simulink model "uz_codegen"  (R2021a)
settings: Solver=VariableStepAuto  StartTime=0.0  StopTime=0.1  RelTol=1e-3  EnableMultiTasking=on
PreLoadFcn:
  | uz_setCodegenPaths
model workspace (MATLAB code in the model file):
  | cmdLim = Simulink.Parameter;
  | cmdLim.Value = 15;
  | cmdLim.Description = 'Limit for controlling the maximum surface command angle.';
  | cmdLim.Min = 0;
  | cmdLim.Max = 90;
  | cmdLim.DocUnits = 'deg';
  | 
  | dispGain = Simulink.Parameter;
  | dispGain.Value = 0.75;
  | dispGain.Description = 'Gain applied to the displacement error.';
  | dispGain.Min = 0;
  | dispGain.Max = [];
  | dispGain.DocUnits = 'deg/sec/deg';
  | 
  | dispLim = Simulink.Parameter;
  | dispLim.Value = 30;
  | dispLim.Description = 'Limit for controlling the maximum commanded angle.';
  | dispLim.Min = 0;
  | dispLim.Max = 180;
  | dispLim.DocUnits = 'deg';
  | 
  | intGain = Simulink.Parameter;
  | intGain.Value = 0.5;
  | intGain.Description = 'Gain applied to the integral error.';
  | intGain.Min = 0;
  | intGain.Max = [];
  | intGain.DocUnits = 'deg/sec/deg/sec';
  | 
  | intLim = Simulink.Parameter;
  | intLim.Value = 5;
  | intLim.Description = 'Limit for controlling the maximum commanded angle.';
  | intLim.Min = 0;
  | intLim.Max = 90;
  | intLim.DocUnits = 'deg';
  | 
  | rateGain = Simulink.Parameter;
  | rateGain.Value = 2;
  | rateGain.Description = 'Gain applied to the rate error.';
  | rateGain.Min = 0;
  | rateGain.Max = [];
  | rateGain.DocUnits = 'deg/deg/sec';
  | 
  | rateLim = Simulink.Parameter;
  | rateLim.Value = 6;
  | rateLim.Description = 'Limit for controlling the maximum commanded angle.';
  | rateLim.Min = 0;
  | rateLim.Max = 180;
  | rateLim.DocUnits = 'deg/sec';
  | 
  | hdgGain = Simulink.Parameter;
  | hdgGain.Value = 0.015;
values from neighbouring files (symbols this model uses):
  f_switchingInverter = 20000    [PMSM_01_Parameter.m]
  Ki_IdController = Kp_IdController * Ki_IdController    (= 100.530964915)    [PMSM_01_Parameter.m]
  Ki_IqController = Kp_IqController * Ki_IqController    (= 100.530964915)    [PMSM_01_Parameter.m]
  Kp_IdController = Kp_IdController    (= 0.0402123859659)    [PMSM_01_Parameter.m]
  Kp_IqController = Kp_IqController    (= 0.0402123859659)    [PMSM_01_Parameter.m]
  Ld = Lq    (= 1.6e-05)    [PMSM_01_Parameter.m]
  Lq = 16e-6    (= 1.6e-05)    [PMSM_01_Parameter.m]
  psi_pm = 0.0048    [PMSM_01_Parameter.m]
  T_controller = 1/f_CurrentController    (= 5e-05)    [PMSM_01_Parameter.m]
  T_dead = 0.2e-10    (= 2e-11)    [PMSM_01_Parameter.m]
  U_DC = 46    [PMSM_01_Parameter.m]
  zp = 21    [PMSM_01_Parameter.m]
undefined symbols (not defined in the file or in its folder): DiscIntNeverNeededParam, U_maxDQ
libraries: nesl_utility x17, ee_lib x15, fl_lib x13, simulink x7, dspsrcs4 x3, pid_lib x2, spsTriangleGeneratorLib x1, spsabctodq0Lib x1, spsdq0toabcLib x1, spsdq0toAlphaBetaZeroLib x1, embmathops x1
(part 2 of 2)

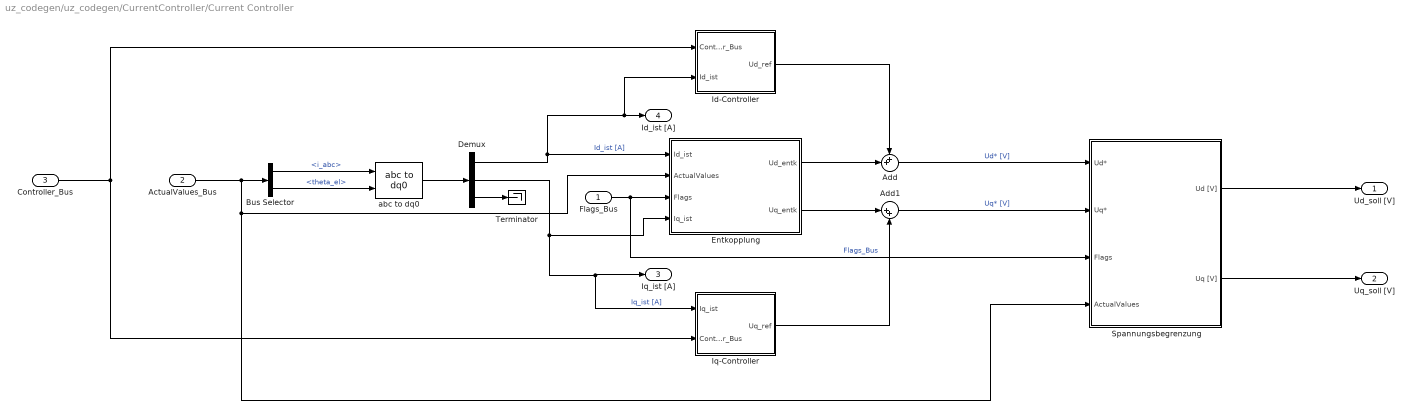
== system uz_codegen/uz_codegen/CurrentController/Current Controller ==
  Flags_Bus : Inport
  ActualValues_Bus : Inport  Port=2
  Controller_Bus : Inport  Port=3
  Add : Sum  Inputs=++|
  Add1 : Sum  Inputs=|++
  Bus Selector : BusSelector  OutputSignals=i_abc,theta_el
  Demux : Demux  Outputs=3
  Entkopplung : Subsystem
  Id-Controller : Subsystem
  Iq-Controller : Subsystem
  Spannungsbegrenzung : Subsystem
  Terminator : Terminator
  abc to dq0 : spsabctodq0Lib/abc to dq0  Alignment=Aligned with phase A axis
  Ud_soll [V] : Outport
  Uq_soll [V] : Outport  Port=2
  Iq_ist [A] : Outport  Port=3
  Id_ist [A] : Outport  Port=4
  wires:
  Add1/1 -> Spannungsbegrenzung/2(Uq*)  "Uq* [V]"
  Add/1 -> Spannungsbegrenzung/1(Ud*)  "Ud* [V]"
  abc to dq0/1 -> Demux/1
  Demux/1 -> Entkopplung/1(Id_ist), Id-Controller/2(Id_ist), Id_ist [A]/1  "Id_ist [A]"
  Demux/2 -> Entkopplung/4(Iq_ist), Iq_ist [A]/1, Iq-Controller/1(Iq_ist)  "Iq_ist [A]"
  Demux/3 -> Terminator/1
  Iq-Controller/1(Uq_ref) -> Add1/2
  Entkopplung/1(Ud_entk) -> Add/2
  Entkopplung/2(Uq_entk) -> Add1/1
  Id-Controller/1(Ud_ref) -> Add/1
  Spannungsbegrenzung/1(Ud [V]) -> Ud_soll [V]/1
  Spannungsbegrenzung/2(Uq [V]) -> Uq_soll [V]/1
  Controller_Bus/1 -> Id-Controller/1(Controller_Bus), Iq-Controller/2(Controller_Bus)
  Bus Selector/1 -> abc to dq0/1  "<i_abc>"
  Bus Selector/2 -> abc to dq0/2  "<theta_el>"
  ActualValues_Bus/1 -> Spannungsbegrenzung/4(ActualValues), Entkopplung/2(ActualValues), Bus Selector/1
  Flags_Bus/1 -> Spannungsbegrenzung/3(Flags), Entkopplung/3(Flags)  "Flags_Bus"

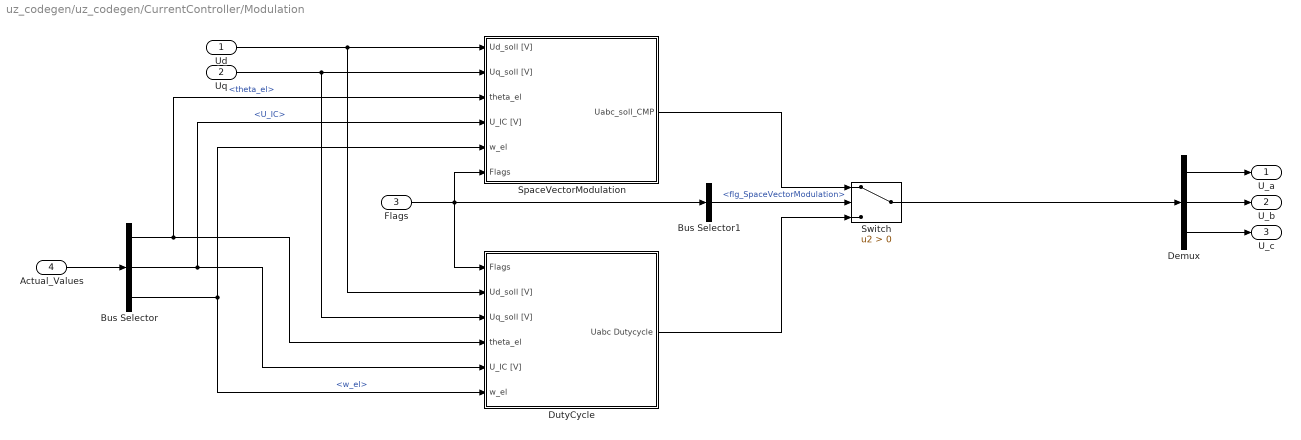
== system uz_codegen/uz_codegen/CurrentController/Modulation ==
  Ud : Inport
  Uq : Inport  Port=2
  Flags : Inport  Port=3
  Actual_Values : Inport  Port=4
  Bus Selector : BusSelector  OutputSignals=theta_el,U_IC,w_el
  Bus Selector1 : BusSelector  OutputSignals=flg_SpaceVectorModulation
  Demux : Demux  Outputs=3
  DutyCycle : Subsystem
  SpaceVectorModulation : Subsystem
  Switch : Switch  Criteria=u2 > Threshold
  U_a : Outport
  U_b : Outport  Port=2
  U_c : Outport  Port=3
  wires:
  Demux/2 -> U_b/1
  Bus Selector1/1 -> Switch/2  "<flg_SpaceVectorModulation>"
  Demux/3 -> U_c/1
  Demux/1 -> U_a/1
  Switch/1 -> Demux/1
  Ud/1 -> DutyCycle/2(Ud_soll [V]), SpaceVectorModulation/1(Ud_soll [V])
  Uq/1 -> DutyCycle/3(Uq_soll [V]), SpaceVectorModulation/2(Uq_soll [V])
  Actual_Values/1 -> Bus Selector/1
  Bus Selector/1 -> DutyCycle/4(theta_el), SpaceVectorModulation/3(theta_el)  "<theta_el>"
  Bus Selector/2 -> DutyCycle/5(U_IC [V]), SpaceVectorModulation/4(U_IC [V])  "<U_IC>"
  Bus Selector/3 -> DutyCycle/6(w_el), SpaceVectorModulation/5(w_el)  "<w_el>"
  DutyCycle/1(Uabc Dutycycle) -> Switch/3
  SpaceVectorModulation/1(Uabc_soll_CMP) -> Switch/1
  Flags/1 -> SpaceVectorModulation/6(Flags), DutyCycle/1(Flags), Bus Selector1/1

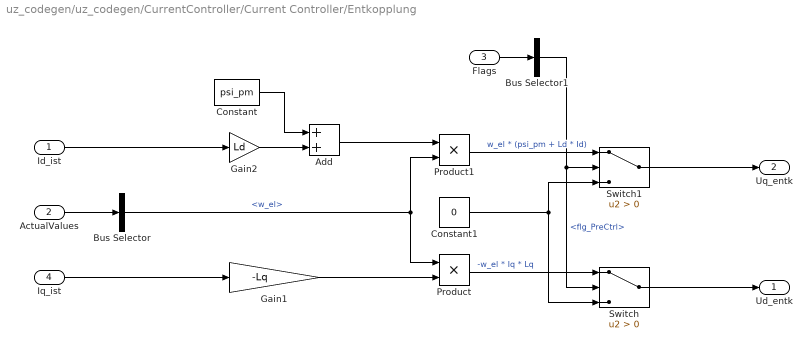
== system uz_codegen/uz_codegen/CurrentController/Current Controller/Entkopplung ==
  Id_ist : Inport
  ActualValues : Inport  Port=2
  Flags : Inport  Port=3
  Iq_ist : Inport  Port=4
  Add : Sum
  Bus Selector : BusSelector  OutputSignals=w_el
  Bus Selector1 : BusSelector  OutputSignals=flg_PreCtrl
  Constant : Constant  Value=psi_pm
  Constant1 : Constant  Value=0
  Gain1 : Gain  Gain=-Lq
  Gain2 : Gain  Gain=Ld
  Product : Product
  Product1 : Product
  Switch : Switch  Criteria=u2 > Threshold
  Switch1 : Switch  Criteria=u2 > Threshold
  Ud_entk : Outport
  Uq_entk : Outport  Port=2
  wires:
  Bus Selector/1 -> Product1/2, Product/1  "<w_el>"
  Iq_ist/1 -> Gain1/1
  Gain1/1 -> Product/2
  Product/1 -> Switch/1  "-w_el * Iq * Lq"
  Id_ist/1 -> Gain2/1
  Gain2/1 -> Add/2
  Constant/1 -> Add/1
  Add/1 -> Product1/1
  Product1/1 -> Switch1/1  "w_el * (psi_pm + Ld * Id)"
  Switch/1 -> Ud_entk/1
  Switch1/1 -> Uq_entk/1
  Constant1/1 -> Switch1/3, Switch/3
  Flags/1 -> Bus Selector1/1
  Bus Selector1/1 -> Switch1/2, Switch/2  "<flg_PreCtrl>"
  ActualValues/1 -> Bus Selector/1

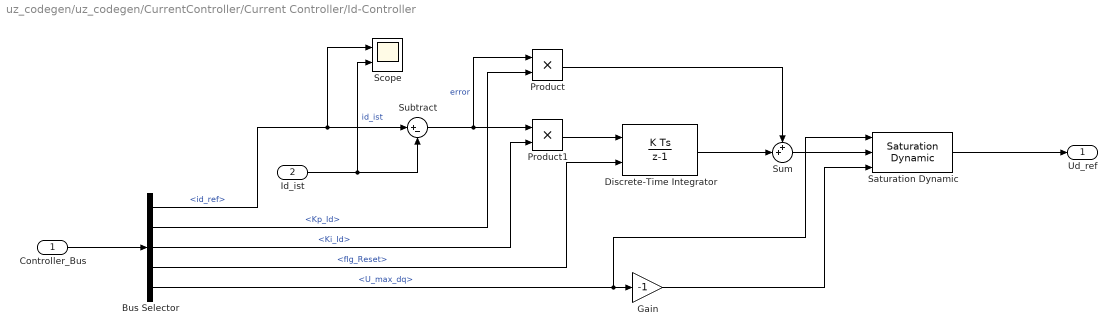
== system uz_codegen/uz_codegen/CurrentController/Current Controller/Id-Controller ==
  Controller_Bus : Inport
  Id_ist : Inport  Port=2
  Bus Selector : BusSelector  OutputSignals=id_ref,Kp_Id,Ki_Id,flg_Reset,U_max_dq
  Discrete-Time Integrator : DiscreteIntegrator  ExternalReset=level  SampleTime=-1  ICPrevOutput=DiscIntNeverNeededParam  ICPrevScaledInput=DiscIntNeverNeededParam
  Gain : Gain  Gain=-1
  Product : Product
  Product1 : Product
  Saturation Dynamic : simulink/Discontinuities/Saturation Dynamic  OutMin=[]  OutMax=[]  OutDataTypeStr=Inherit: Same as second input  OutDataType=fixdt(1, 16)  OutScaling=2^-10  DoSatur=off
  Scope : Scope  NumInputPorts=2
  Subtract : Sum  Inputs=|+-
  Sum : Sum  Inputs=++|
  Ud_ref : Outport
  wires:
  Bus Selector/1 -> Scope/1, Subtract/1  "<id_ref>"
  Gain/1 -> Saturation Dynamic/3
  Bus Selector/2 -> Product/2  "<Kp_Id>"
  Bus Selector/4 -> Discrete-Time Integrator/2  "<flg_Reset>"
  Id_ist/1 -> Subtract/2, Scope/2  "id_ist"
  Bus Selector/3 -> Product1/2  "<Ki_Id>"
  Controller_Bus/1 -> Bus Selector/1
  Bus Selector/5 -> Saturation Dynamic/1, Gain/1  "<U_max_dq>"
  Sum/1 -> Saturation Dynamic/2
  Saturation Dynamic/1 -> Ud_ref/1
  Product/1 -> Sum/1
  Subtract/1 -> Product/1, Product1/1  "error"
  Discrete-Time Integrator/1 -> Sum/2
  Product1/1 -> Discrete-Time Integrator/1

== system uz_codegen/uz_codegen/CurrentController/Current Controller/Iq-Controller ==
  Iq_ist : Inport
  Controller_Bus : Inport  Port=2
  Bus Selector : BusSelector  OutputSignals=iq_ref,Kp_Iq,Ki_Iq,flg_Reset,U_max_dq
  Discrete-Time Integrator : DiscreteIntegrator  ExternalReset=level  SampleTime=-1  ICPrevOutput=DiscIntNeverNeededParam  ICPrevScaledInput=DiscIntNeverNeededParam
  Gain : Gain  Gain=-1
  Product : Product
  Product1 : Product
  Saturation Dynamic : simulink/Discontinuities/Saturation Dynamic  OutMin=[]  OutMax=[]  OutDataTypeStr=Inherit: Same as second input  OutDataType=fixdt(1, 16)  OutScaling=2^-10  DoSatur=off
  Scope : Scope  NumInputPorts=2
  Subtract : Sum  Inputs=|+-
  Sum : Sum  Inputs=++|
  Uq_ref : Outport
  wires:
  Iq_ist/1 -> Subtract/2, Scope/2  "iq_ist"
  Controller_Bus/1 -> Bus Selector/1
  Bus Selector/2 -> Product/2  "<Kp_Iq>"
  Bus Selector/3 -> Product1/2  "<Ki_Iq>"
  Bus Selector/4 -> Discrete-Time Integrator/2  "<flg_Reset>"
  Bus Selector/5 -> Saturation Dynamic/1, Gain/1  "<U_max_dq>"
  Gain/1 -> Saturation Dynamic/3
  Bus Selector/1 -> Scope/1, Subtract/1  "<iq_ref>"
  Subtract/1 -> Product/1, Product1/1  "error"
  Product1/1 -> Discrete-Time Integrator/1
  Discrete-Time Integrator/1 -> Sum/2
  Product/1 -> Sum/1
  Sum/1 -> Saturation Dynamic/2
  Saturation Dynamic/1 -> Uq_ref/1

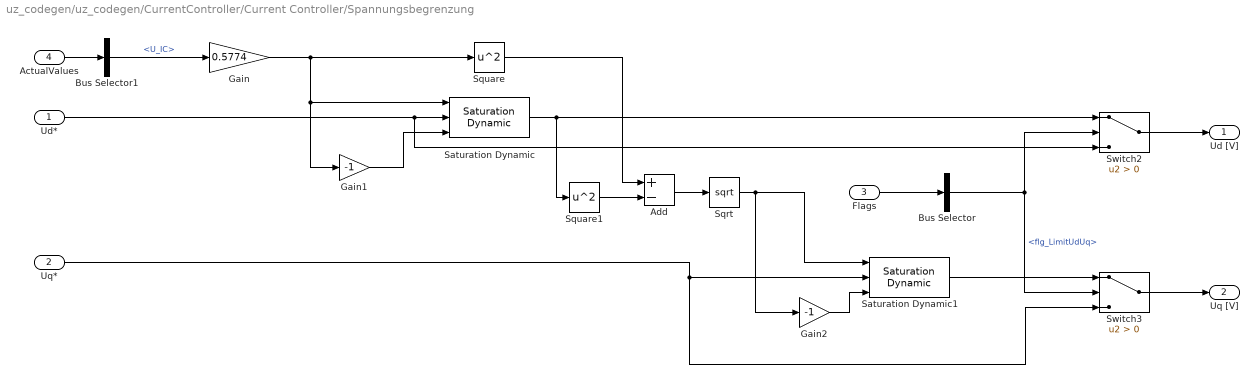
== system uz_codegen/uz_codegen/CurrentController/Current Controller/Spannungsbegrenzung ==
  Ud* : Inport
  Uq* : Inport  Port=2
  Flags : Inport  Port=3
  ActualValues : Inport  Port=4
  Add : Sum  Inputs=+-
  Bus Selector : BusSelector  OutputSignals=flg_LimitUdUq
  Bus Selector1 : BusSelector  OutputSignals=U_IC
  Gain : Gain  Gain=0.5774
  Gain1 : Gain  Gain=-1
  Gain2 : Gain  Gain=-1
  Saturation Dynamic : simulink/Discontinuities/Saturation Dynamic  OutMin=[]  OutMax=[]  OutDataTypeStr=Inherit: Same as second input  OutDataType=fixdt(1, 16)  OutScaling=2^-10  DoSatur=off
  Saturation Dynamic1 : simulink/Discontinuities/Saturation Dynamic  OutMin=[]  OutMax=[]  OutDataTypeStr=Inherit: Same as second input  OutDataType=fixdt(1, 16)  OutScaling=2^-10  DoSatur=off
  Sqrt : Sqrt  SaturateOnIntegerOverflow=on
  Square : Math  Operator=square  SaturateOnIntegerOverflow=on
  Square1 : Math  Operator=square  SaturateOnIntegerOverflow=on
  Switch2 : Switch  Criteria=u2 > Threshold
  Switch3 : Switch  Criteria=u2 > Threshold
  Ud [V] : Outport
  Uq [V] : Outport  Port=2
  wires:
  Gain2/1 -> Saturation Dynamic1/3
  Add/1 -> Sqrt/1
  Square/1 -> Add/1
  Sqrt/1 -> Gain2/1, Saturation Dynamic1/1
  Saturation Dynamic/1 -> Switch2/1, Square1/1
  Gain1/1 -> Saturation Dynamic/3
  Uq*/1 -> Saturation Dynamic1/2, Switch3/3
  Bus Selector1/1 -> Gain/1  "<U_IC>"
  Gain/1 -> Square/1, Saturation Dynamic/1, Gain1/1
  Square1/1 -> Add/2
  Ud*/1 -> Saturation Dynamic/2, Switch2/3
  Switch3/1 -> Uq [V]/1
  Switch2/1 -> Ud [V]/1
  Saturation Dynamic1/1 -> Switch3/1
  Flags/1 -> Bus Selector/1
  Bus Selector/1 -> Switch3/2, Switch2/2  "<flg_LimitUdUq>"
  ActualValues/1 -> Bus Selector1/1

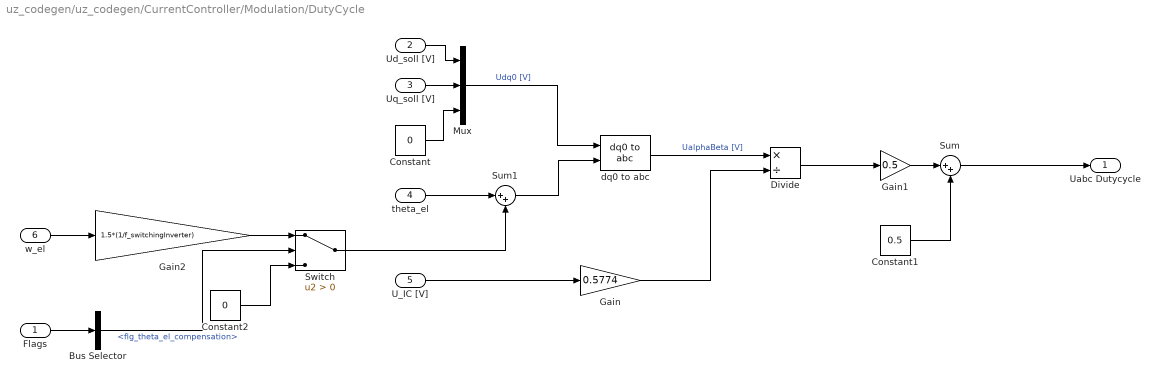
== system uz_codegen/uz_codegen/CurrentController/Modulation/DutyCycle ==
  Flags : Inport
  Ud_soll [V] : Inport  Port=2
  Uq_soll [V] : Inport  Port=3
  theta_el : Inport  Port=4
  U_IC [V] : Inport  Port=5
  w_el : Inport  Port=6
  Bus Selector : BusSelector  OutputSignals=flg_theta_el_compensation
  Constant : Constant  Value=0
  Constant1 : Constant  Value=0.5
  Constant2 : Constant  Value=0
  Divide : Product  Inputs=*/
  Gain : Gain  Gain=0.5774
  Gain1 : Gain  Gain=0.5
  Gain2 : Gain  Gain=1.5*(1/f_switchingInverter)
  Mux : Mux  Inputs=3
  Sum : Sum  Inputs=|++
  Sum1 : Sum  Inputs=|++
  Switch : Switch  Criteria=u2 > Threshold
  dq0 to abc : spsdq0toabcLib/dq0 to abc  Alignment=Aligned with phase A axis
  Uabc Dutycycle : Outport
  wires:
  Constant/1 -> Mux/3
  U_IC [V]/1 -> Gain/1
  dq0 to abc/1 -> Divide/1  "UalphaBeta [V]"
  Mux/1 -> dq0 to abc/1  "Udq0 [V]"
  Uq_soll [V]/1 -> Mux/2
  Ud_soll [V]/1 -> Mux/1
  theta_el/1 -> Sum1/1
  Gain/1 -> Divide/2
  Divide/1 -> Gain1/1
  Gain1/1 -> Sum/1
  Constant1/1 -> Sum/2
  Sum/1 -> Uabc Dutycycle/1
  Sum1/1 -> dq0 to abc/2
  w_el/1 -> Gain2/1
  Gain2/1 -> Switch/1
  Switch/1 -> Sum1/2
  Constant2/1 -> Switch/3
  Flags/1 -> Bus Selector/1
  Bus Selector/1 -> Switch/2  "<flg_theta_el_compensation>"

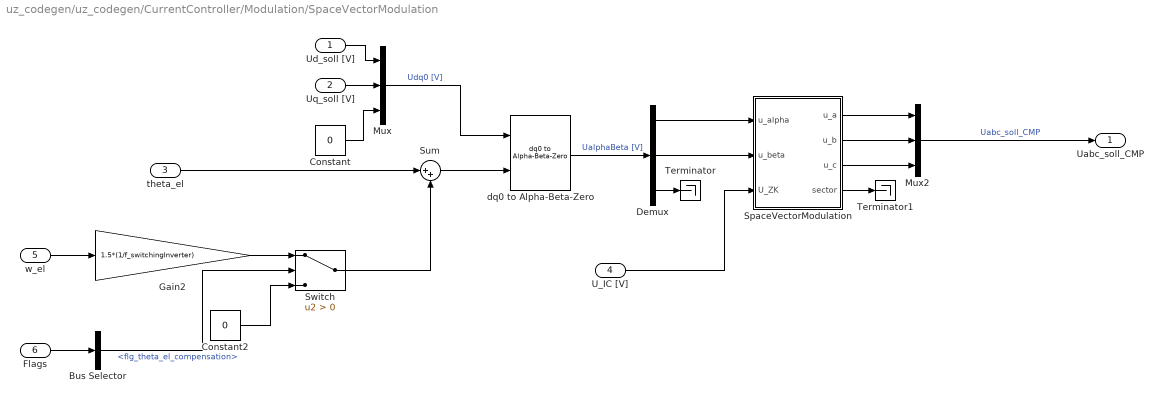
== system uz_codegen/uz_codegen/CurrentController/Modulation/SpaceVectorModulation ==
  Ud_soll [V] : Inport
  Uq_soll [V] : Inport  Port=2
  theta_el : Inport  Port=3
  U_IC [V] : Inport  Port=4
  w_el : Inport  Port=5
  Flags : Inport  Port=6
  Bus Selector : BusSelector  OutputSignals=flg_theta_el_compensation
  Constant : Constant  Value=0
  Constant2 : Constant  Value=0
  Demux : Demux  Outputs=3
  Gain2 : Gain  Gain=1.5*(1/f_switchingInverter)
  Mux : Mux  Inputs=3
  Mux2 : Mux  Inputs=3
  SpaceVectorModulation : MATLAB Function  TreatAsAtomicUnit=on
  Sum : Sum  Inputs=|++
  Switch : Switch  Criteria=u2 > Threshold
  Terminator : Terminator
  Terminator1 : Terminator
  dq0 to Alpha-Beta-Zero : spsdq0toAlphaBetaZeroLib/dq0 to Alpha-Beta-Zero  Alignment=Aligned with phase A axis
      settings: SourceProductBaseCode=PS
  Uabc_soll_CMP : Outport
  wires:
  Ud_soll [V]/1 -> Mux/1
  Uq_soll [V]/1 -> Mux/2
  Constant/1 -> Mux/3
  Mux/1 -> dq0 to Alpha-Beta-Zero/1  "Udq0 [V]"
  theta_el/1 -> Sum/1
  Demux/1 -> SpaceVectorModulation/1(u_alpha)
  Demux/2 -> SpaceVectorModulation/2(u_beta)
  Demux/3 -> Terminator/1
  SpaceVectorModulation/1(u_a) -> Mux2/1
  SpaceVectorModulation/2(u_b) -> Mux2/2
  SpaceVectorModulation/3(u_c) -> Mux2/3
  dq0 to Alpha-Beta-Zero/1 -> Demux/1  "UalphaBeta [V]"
  Mux2/1 -> Uabc_soll_CMP/1  "Uabc_soll_CMP"
  U_IC [V]/1 -> SpaceVectorModulation/3(U_ZK)
  SpaceVectorModulation/4(sector) -> Terminator1/1
  w_el/1 -> Gain2/1
  Constant2/1 -> Switch/3
  Flags/1 -> Bus Selector/1
  Gain2/1 -> Switch/1
  Bus Selector/1 -> Switch/2  "<flg_theta_el_compensation>"
  Sum/1 -> dq0 to Alpha-Beta-Zero/2
  Switch/1 -> Sum/2

== stateflow chart uz_codegen/uz_codegen ==
  settings: updateMethod=DISCRETE  sampleTime=T_controller
  state Start
    entry:
    activeState = 1;
    Ua_DutyCycle = 0;
    Ub_DutyCycle = 0;
    Uc_DutyCycle = 0;
  state Reset
    during:
    activeState = 3;
    [Ua_DutyCycle, Ub_DutyCycle, Uc_DutyCycle, iq_ist, id_ist, ud, uq] = CurrentController(ia, ib, ic, w_el, flg_PreCntr, theta_el, U_IC,id_ref,iq_ref,flgLimitUdUq, Kp_Iq, Ki_Iq, Kp_Id, Ki_Id, flg_SpaceVectorModulation, RESET, flg_deadTimeCompensation, flg_theta_el_compensation)
    Ua_DutyCycle = 0;
    Ub_DutyCycle = 0;
    Uc_DutyCycle = 0;
  state InProcess
    entry:
    activeState = 2;
    during:
    [Ua_DutyCycle, Ub_DutyCycle, Uc_DutyCycle, iq_ist, id_ist, ud, uq] = CurrentController(ia, ib, ic, w_el, flg_PreCntr, theta_el, U_IC,id_ref,iq_ref,flgLimitUdUq, Kp_Iq, Ki_Iq, Kp_Id, Ki_Id, flg_SpaceVectorModulation, RESET, flg_deadTimeCompensation, flg_theta_el_compensation)
  state [ua,ub,uc,Iq_ist,Id_ist,ud_soll,uq_soll] = CurrentController(ia,ib,ic,w_el,flg_PreCtrl,theta_el,U_IC,id_ref,iq_ref,flg_LimitUdUq,Kp_Iq,Ki_Iq,Kp_Id,Ki_Id,flg_SpaceVectorModulation,flg_Reset,flg_deadTimeCompensation, flg_theta_el_compensation) [function]
  (default) -> Start
  Reset -> Start : [RESET == 0]
  InProcess -> Reset : [RESET==1]
  Start -> InProcess : [START==1 & RESET==0]
  data: ia function_input double size=1; ib function_input double size=1; ic function_input double size=1; w_el function_input double size=1; flg_PreCtrl function_input double size=1; theta_el function_input double size=1; ua function_output; ub function_output; uc function_output; Iq_ist function_output; Id_ist function_output; ud_soll function_output; uq_soll function_output; U_IC function_input double size=1; id_ref function_input double size=1; iq_ref function_input double size=1; flg_LimitUdUq function_input double size=1; Kp_Iq function_input double size=1; Ki_Iq function_input double size=1; Kp_Id function_input double size=1; Ki_Id function_input double size=1; flg_SpaceVectorModulation function_input double size=1; flg_Reset function_input double size=1; flg_deadTimeCompensation function_input double size=1; flg_theta_el_compensation function_input double size=1; flg_PreCntr input; ic input; ib input; w_el input; ia input; theta_el input; iq_ref input; id_ref input; Ua_DutyCycle output; activeState output; Uc_DutyCycle output; Ub_DutyCycle output; iq_ist output; id_ist output; U_IC input; RESET input; START input; uq output; ud output; flgLimitUdUq input; flg_SpaceVectorModulation input; Kp_Iq input; Kp_Id input; Ki_Iq input; Ki_Id input; flg_deadTimeCompensation input; flg_theta_el_compensation input

== matlab function uz_codegen/CurrentController/Modulation/SpaceVectorModulation/SpaceVectorModulation ==
  data: u_alpha input; u_a output; u_beta input; U_ZK input; u_b output; u_c output; sector output
function [u_a, u_b, u_c, sector] = fcn(u_alpha, u_beta, U_ZK)

a_U_on=0;
a_V_on=0;
a_W_on=0;

 %%__%%__%%__%%__%%__%%__%%__%%__%%__%%__%%__%%__%%__%%__%%__%%__%%__%%__%%_
    %%Trägerbasierte Raumzeigermodulation%%
    %%Eingänge:
    %U_ZK       -- Zwischenkreisspannung
    %u_alpha    -- alphakomponente des Sollspannungsraumzeigers
    %u_beta     -- betakomponente des Sollspannungsraumzeigers
    %CMP_Period_max_val  -- maximalwert des Dreiecks/Sägezahnzählers zum Gewichten der Aussteuergrade
    %%Ausgänge:
    %CMP_U        -- Vergleichswert U
    %CMP_V        -- Vergleichswert V
    %CMP_W        -- Vergleichswert W
    %sector       -- Ausgabe des Sektors des Spannungszeigers
    
    
    %Berechnung von a, b, c nach Quang Dittrich S24
    
    a = abs(u_alpha) + 0.5774*abs(u_beta);
    b = abs(u_alpha) - 0.5774*abs(u_beta);
    c = 1.1547*abs(u_beta);
    
    U_max = 0.6667 * U_ZK; %Maximum Voltage U_ZL/sqrt(3)
    
    
    %Sektor und Quadranten nach Quang Dittrich S32
    if(u_beta < 0)
        if (u_alpha <0)
            quadrant=3;
            if(b < 0)
                sector = 5;
            else
                sector = 4;
            end
        else
            quadrant=4;
            if(b < 0)
                sector = 5;
            else
                sector = 6;
            end
        end
        
    else
        if (u_alpha <0)
            quadrant=2;
            if(b < 0)
                sector = 2;
            else
                sector = 3;
            end
        else
            quadrant=1;
            if(b < 0)
                sector = 2;
            else
                sector = 1;
            end
        end
    end
    
    sector = sector;
    
    %%Modulationsfunktionen für Phasen U,V,W
    %%Erzeugung der Aussteuergrade für die Halbbrücken
    %%--> Erzeugung einer "regulary Sampled SVM" erfolgt anschließend durch Abtastung
    %%mit Dreieckszählern in Hardware.
    
    if (sector == 1)
        
        %Quang S.24 and normed to 2/3 U_DC
        u1 = b/(U_max);
        u2 = c/(U_max);
        
        %Quang S.34
        a_U_on = 0.5 + u1*0.5 + u2*0.5;
        a_V_on = 0.5 - u1*0.5 + u2*0.5;
        a_W_on = 0.5 - u1*0.5 - u2*0.5;
    end
    
    
    if ((sector == 2) && (quadrant == 1))
        
        u1 = a/(U_max);
        u2 = (-abs(u_alpha) + 0.5774*abs(u_beta))/(U_max);
        
        a_U_on = 0.5 + u1*0.5 - u2*0.5;
        a_V_on = 0.5 + u1*0.5 + u2*0.5;
        a_W_on = 0.5 - u1*0.5 - u2*0.5;
    end
    
    
    if ((sector == 2) && (quadrant == 2))
        
        u1 = (-abs(u_alpha) + 0.5774*abs(u_beta))/(U_max);
        u2 = a/(U_max);
        
        a_U_on = 0.5 + u1*0.5 - u2*0.5;
        a_V_on = 0.5 + u1*0.5 + u2*0.5;
        a_W_on = 0.5 - u1*0.5 - u2*0.5;
    end
    
    
    if (sector == 3)
        
        u1 = c/(U_max);
        u2 = b/(U_max);
        
        a_U_on=  0.5 - u1*0.5 - u2*0.5;
        a_V_on = 0.5 + u1*0.5 + u2*0.5;
        a_W_on = 0.5 - u1*0.5 + u2*0.5;
    end
    
    if (sector == 4)
        
        u1 = b/(U_max);
        u2 = c/(U_max);
        
        a_U_on = 0.5 - u1*0.5 - u2*0.5;
        a_V_on = 0.5 + u1*0.5 - u2*0.5;
        a_W_on = 0.5 + u1*0.5 + u2*0.5;
    end
    
    
    if ((sector == 5) && (quadrant == 3))
        
        u1 = a/(U_max);
        u2 = (-abs(u_alpha) + 0.5774*abs(u_beta))/(U_max);
        
        a_U_on = 0.5 - u1*0.5 + u2*0.5;
        a_V_on = 0.5 - u1*0.5 - u2*0.5;
        a_W_on = 0.5 + u1*0.5 + u2*0.5;
    end
    
    
    if ((sector == 5) && (quadrant == 4))
        
        u1 =(-abs(u_alpha) + 0.5774*abs(u_beta))/(U_max);
        u2 =  a/(U_max);
        
        a_U_on = 0.5 - u1*0.5 + u2*0.5;
        a_V_on = 0.5 - u1*0.5 - u2*0.5;
        a_W_on = 0.5 + u1*0.5 + u2*0.5;
    end
    
    
    if (sector == 6)
        
        u1 = c/(U_max);
        u2 = b/(U_max);
        
        a_U_on = 0.5 + u1*0.5 + u2*0.5;
        a_V_on = 0.5 - u1*0.5 - u2*0.5;
        a_W_on = 0.5 + u1*0.5 - u2*0.5;
    end
    
    if a_U_on > 1.0
        a_U_on = 1.0;
    end
    if a_V_on > 1.0
        a_V_on = 1.0;
    end
    if a_W_on > 1.0
        a_W_on = 1.0;
    end     
        
    u_a = a_U_on;
    u_b = a_V_on;
    u_c = a_W_on;
